simulink model "phase_comp"  (Simulink 5.0)
settings: Solver=ode45  StartTime=0.0  StopTime=10  RelTol=1e-3
values from neighbouring files (symbols this model uses):
  A = [[-1/C1*(1/Ri+1/Rth)      1/C1/Ri           0   ] ... (first row only)    [pll_init_2.m]
  B = [[1/C1 0 0].' [1/C1/Rth 0 0].']    [pll_init_2.m]
  C = [0 1 0]    [pll_init_2.m]
  Cvc1 = [1 0 0]    [pll_init_2.m]
  fvcxo = 148.5e6/1.001    (= 148351648.352)    [pll_init_2.m]
  Kvcxo = 90e-6    (= 9e-05)    [pll_init_2.m]
  Ndec1 = 91    [pll_init_2.m]
  Ndec2 = 500    [pll_init_2.m]
  R1 = 7700    [Phase_comp_init.m]    (also in pll_init_2.m = 220)
  R2 = 4700    [Phase_comp_init.m]    (also in pll_init_2.m = 220)
  t_both = 5e-9    (= 5e-09)    [Phase_comp_init.m]    (also in pll_init_2.m = 2e-09)
  Tpll = 1/300000    (= 3.33333333333e-06)    [Phase_comp_init.m]    (also in pll_init_2.m = 3.37037037037e-06)
  Vcc = 3.3    [Phase_comp_init.m]    (also in pll_init_2.m)
  Vvcxo0 = 1.25    [pll_init_2.m]
  Vvcxomax = 2.5    [pll_init_2.m]
  Vvcxomin = 0    [pll_init_2.m]
libraries: simulink x4
settings Model: LastModifiedBy=thh

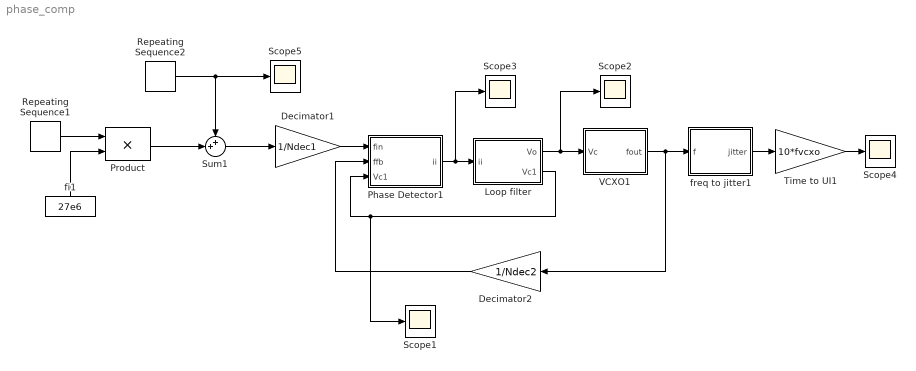
== system phase_comp ==
  Decimator1 : Gain  Gain=1/Ndec1  SaturateOnIntegerOverflow=on
  Decimator2 : Gain  Orientation=left  Gain=1/Ndec2  SaturateOnIntegerOverflow=on
  Loop filter : Subsystem
  Phase Detector1 : Subsystem
  Product : Product  SaturateOnIntegerOverflow=on
  Repeating Sequence1 : simulink/Sources/Repeating Sequence  rep_seq_t=[0 10 10 20]  rep_seq_y=1+([0 0 30 30]*1e-6)*0
  Repeating Sequence2 : simulink/Sources/Repeating Sequence  rep_seq_t=[0 8-1e-3 8-1e-3 8 8 16-1e-3 16-1e-3 16]  rep_seq_y=[0 0 1 1 0 0 -1 -1]*30*1e3
  Scope{1..5} (5 alike) : Scope
      Scope1 settings: TimeRange=10  YMin=-0.5  YMax=3.5
      Scope2 settings: TimeRange=10  YMin=1.25  YMax=1.25025  SaveName=ScopeData3
      Scope3 settings: TimeRange=10  YMin=-0.0001  YMax=0.0012  SaveName=ScopeData5
      Scope4 settings: TimeRange=13.94281180037974  YMin=15  YMax=27  SaveName=ScopeData4
      Scope5 settings: TimeRange=13.94281180037974  YMin=-1  YMax=1  SaveName=ScopeData2
  Sum1 : Sum  Inputs=++|  SaturateOnIntegerOverflow=on
  Time to UI1 : Gain  Gain=10*fvcxo  SaturateOnIntegerOverflow=on
  VCXO1 : Subsystem
  fi1 : Constant  Orientation=up  Value=27e6
  freq to jitter1 : Subsystem
  wires:
  freq to jitter1/1(jitter) -> Time to UI1/1
  Time to UI1/1 -> Scope4/1
  VCXO1/1(fout) -> freq to jitter1/1(f), Decimator2/1
  Decimator2/1 -> Phase Detector1/2(ffb)
  fi1/1 -> Product/2
  Repeating Sequence1/1 -> Product/1
  Phase Detector1/1(ii) -> Loop filter/1(ii), Scope3/1
  Decimator1/1 -> Phase Detector1/1(fin)
  Repeating Sequence2/1 -> Sum1/1, Scope5/1
  Product/1 -> Sum1/2
  Sum1/1 -> Decimator1/1
  Loop filter/2(Vc1) -> Phase Detector1/3(Vc1), Scope1/1
  Loop filter/1(Vo) -> VCXO1/1(Vc), Scope2/1

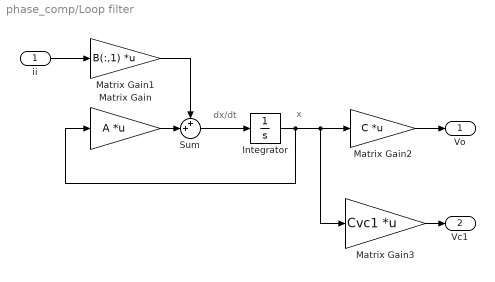
== system phase_comp/Loop filter ==
  note: x
  note: dx/dt
  ii : Inport
  Integrator : Integrator  InitialCondition=Vvcxo0*[1 1 1].'
  Matrix Gain : Gain  Gain=A  Multiplication=Matrix(K*u) (u vector)  SaturateOnIntegerOverflow=on
  Matrix Gain1 : Gain  Gain=B(:,1)  Multiplication=Matrix(K*u)  SaturateOnIntegerOverflow=on
  Matrix Gain2 : Gain  Gain=C  Multiplication=Matrix(K*u) (u vector)  SaturateOnIntegerOverflow=on
  Matrix Gain3 : Gain  Gain=Cvc1  Multiplication=Matrix(K*u) (u vector)  SaturateOnIntegerOverflow=on
  Sum : Sum  Inputs=++|  SaturateOnIntegerOverflow=on
  Vo : Outport
  Vc1 : Outport  Port=2
  wires:
  Integrator/1 -> Matrix Gain/1, Matrix Gain2/1, Matrix Gain3/1
  Sum/1 -> Integrator/1
  Matrix Gain/1 -> Sum/2
  Matrix Gain1/1 -> Sum/1
  Matrix Gain2/1 -> Vo/1
  ii/1 -> Matrix Gain1/1
  Matrix Gain3/1 -> Vc1/1

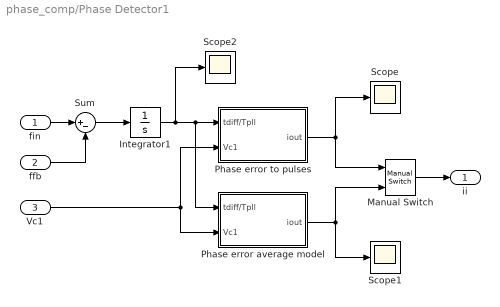
== system phase_comp/Phase Detector1 ==
  fin : Inport
  ffb : Inport  Port=2
  Vc1 : Inport  Port=3
  Integrator1 : Integrator  InitialCondition=0.062
  Manual Switch : simulink/Signal Routing/Manual Switch  sw=0  action=0
  Phase error average model : Subsystem
  Phase error to pulses : Subsystem
  Scope : Scope
      settings: TimeRange=0.001  YMin=-0.2  YMax=1.2  SaveName=ScopeData6
  Scope1 : Scope
      settings: TimeRange=0.001  YMin=-0.000275  YMax=0.0001  SaveName=ScopeData7
  Scope2 : Scope
      settings: TimeRange=0.001  YMin=0.0606  YMax=0.062
  Sum : Sum  Inputs=|+-  SaturateOnIntegerOverflow=on
  ii : Outport
  wires:
  ffb/1 -> Sum/2
  fin/1 -> Sum/1
  Sum/1 -> Integrator1/1
  Manual Switch/1 -> ii/1
  Integrator1/1 -> Phase error to pulses/1(tdiff/Tpll), Phase error average model/1(tdiff/Tpll), Scope2/1
  Phase error to pulses/1(iout) -> Scope/1, Manual Switch/1
  Vc1/1 -> Phase error to pulses/2(Vc1), Phase error average model/2(Vc1)
  Phase error average model/1(iout) -> Scope1/1, Manual Switch/2

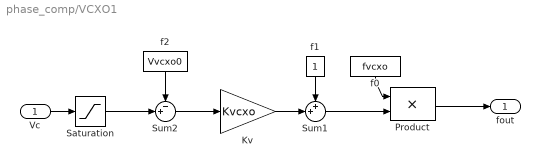
== system phase_comp/VCXO1 ==
  Vc : Inport
  Kv : Gain  Gain=Kvcxo  SaturateOnIntegerOverflow=on
  Product : Product  SaturateOnIntegerOverflow=on
  Saturation : Saturate  UpperLimit=Vvcxomax  LowerLimit=Vvcxomin
  Sum1 : Sum  Inputs=++|  SaturateOnIntegerOverflow=on
  Sum2 : Sum  Inputs=-+|  SaturateOnIntegerOverflow=on
  f0 : Constant  Orientation=down  Value=fvcxo
  f1 : Constant  Orientation=down
  f2 : Constant  Orientation=down  Value=Vvcxo0
  fout : Outport
  wires:
  f2/1 -> Sum2/1
  Vc/1 -> Saturation/1
  Sum2/1 -> Kv/1
  Product/1 -> fout/1
  Kv/1 -> Sum1/2
  Sum1/1 -> Product/2
  f1/1 -> Sum1/1
  f0/1 -> Product/1
  Saturation/1 -> Sum2/2

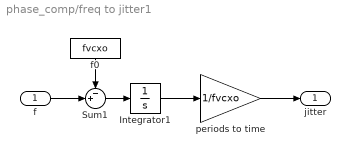
== system phase_comp/freq to jitter1 ==
  f : Inport
  Integrator1 : Integrator
  Sum1 : Sum  Inputs=-+|  SaturateOnIntegerOverflow=on
  f0 : Constant  Orientation=down  Value=fvcxo
  periods to time : Gain  Gain=1/fvcxo  SaturateOnIntegerOverflow=on
  jitter : Outport
  wires:
  periods to time/1 -> jitter/1
  f/1 -> Sum1/2
  f0/1 -> Sum1/1
  Sum1/1 -> Integrator1/1
  Integrator1/1 -> periods to time/1

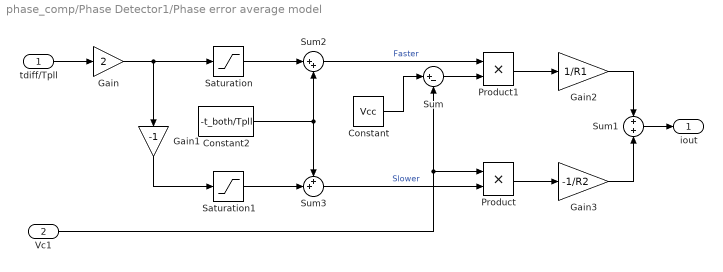
== system phase_comp/Phase Detector1/Phase error average model ==
  tdiff/Tpll : Inport
  Vc1 : Inport  Port=2
  Constant : Constant  Value=Vcc
  Constant2 : Constant  Value=-t_both/Tpll
  Gain : Gain  Gain=2  SaturateOnIntegerOverflow=on
  Gain1 : Gain  Orientation=down  Gain=-1  SaturateOnIntegerOverflow=on
  Gain2 : Gain  Gain=1/R1  SaturateOnIntegerOverflow=on
  Gain3 : Gain  Gain=-1/R2  SaturateOnIntegerOverflow=on
  Product : Product  SaturateOnIntegerOverflow=on
  Product1 : Product  SaturateOnIntegerOverflow=on
  Saturation : Saturate  UpperLimit=1  LowerLimit=0
  Saturation1 : Saturate  UpperLimit=1  LowerLimit=0
  Sum : Sum  Inputs=|+-  SaturateOnIntegerOverflow=on
  Sum1 : Sum  SaturateOnIntegerOverflow=on
  Sum2 : Sum  Inputs=|++  SaturateOnIntegerOverflow=on
  Sum3 : Sum  Inputs=++|  SaturateOnIntegerOverflow=on
  iout : Outport
  wires:
  Product/1 -> Gain3/1
  Sum/1 -> Product1/2
  Sum1/1 -> iout/1
  Gain2/1 -> Sum1/1
  Gain3/1 -> Sum1/2
  Product1/1 -> Gain2/1
  Vc1/1 -> Sum/2, Product/1
  Constant/1 -> Sum/1
  Sum3/1 -> Product/2  "Slower"
  Sum2/1 -> Product1/1  "Faster"
  tdiff/Tpll/1 -> Gain/1
  Gain1/1 -> Saturation1/1
  Saturation1/1 -> Sum3/2
  Gain/1 -> Gain1/1, Saturation/1
  Saturation/1 -> Sum2/1
  Constant2/1 -> Sum2/2, Sum3/1

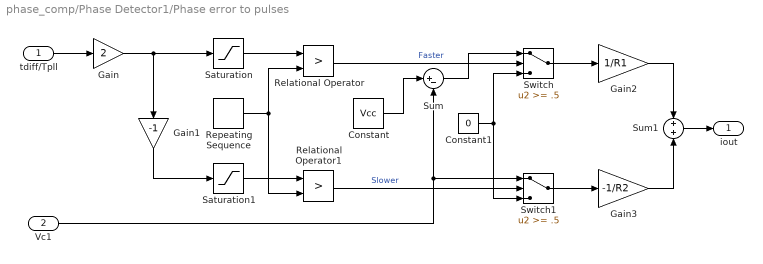
== system phase_comp/Phase Detector1/Phase error to pulses ==
  tdiff/Tpll : Inport
  Vc1 : Inport  Port=2
  Constant : Constant  Value=Vcc
  Constant1 : Constant  Value=0
  Gain : Gain  Gain=2  SaturateOnIntegerOverflow=on
  Gain1 : Gain  Orientation=down  Gain=-1  SaturateOnIntegerOverflow=on
  Gain2 : Gain  Gain=1/R1  SaturateOnIntegerOverflow=on
  Gain3 : Gain  Gain=-1/R2  SaturateOnIntegerOverflow=on
  Relational Operator : RelationalOperator  Operator=>
  Relational Operator1 : RelationalOperator  Operator=>
  Repeating Sequence : simulink/Sources/Repeating Sequence  rep_seq_t=[0 Tpll]  rep_seq_y=[1 0]-t_both/Tpll
  Saturation : Saturate  UpperLimit=1  LowerLimit=0
  Saturation1 : Saturate  UpperLimit=1  LowerLimit=0
  Sum : Sum  Inputs=|+-  SaturateOnIntegerOverflow=on
  Sum1 : Sum  SaturateOnIntegerOverflow=on
  Switch : Switch  Threshold=.5  SaturateOnIntegerOverflow=on
  Switch1 : Switch  Threshold=.5  SaturateOnIntegerOverflow=on
  iout : Outport
  wires:
  Repeating Sequence/1 -> Relational Operator/2, Relational Operator1/2
  Saturation/1 -> Relational Operator/1
  Gain/1 -> Saturation/1, Gain1/1
  Saturation1/1 -> Relational Operator1/1
  Gain1/1 -> Saturation1/1
  tdiff/Tpll/1 -> Gain/1
  Relational Operator/1 -> Switch/2  "Faster"
  Relational Operator1/1 -> Switch1/2  "Slower"
  Constant/1 -> Sum/1
  Vc1/1 -> Sum/2, Switch1/1
  Switch/1 -> Gain2/1
  Gain3/1 -> Sum1/2
  Gain2/1 -> Sum1/1
  Sum1/1 -> iout/1
  Constant1/1 -> Switch/3, Switch1/3
  Sum/1 -> Switch/1
  Switch1/1 -> Gain3/1
